simulink model "lab01_1"  (R2025a)
settings: Solver=VariableStepAuto  StartTime=0.0  StopTime=10  RelTol=1e-3
settings Model: Creator=grigorijtomczuk  LastModifiedBy=grigorijtomczuk

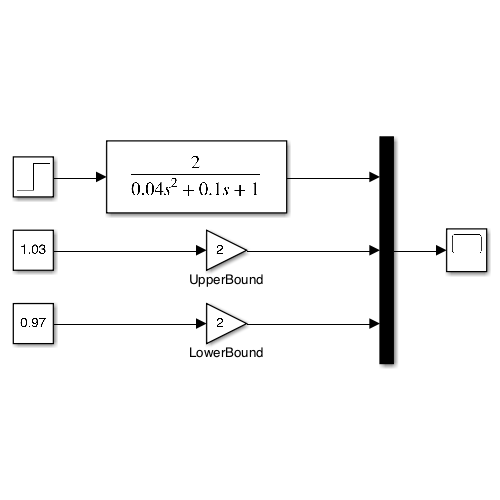
[thumbnail: Simulink's stored preview of the top-level diagram]
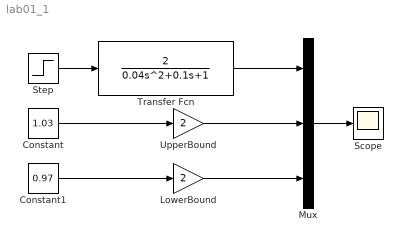
== system lab01_1 ==
  Constant : Constant  Value=1.03
  Constant1 : Constant  Value=0.97
  LowerBound : Gain  Gain=2
  Mux : Mux  Inputs=3
  Scope : Scope
      settings: ActiveDisplayYMinimum=-0.35929013888602573  ActiveDisplayYMaximum=3.2336112499742322
  Step : Step  SampleTime=0
  Transfer Fcn : TransferFcn  Numerator=[2]  Denominator=[0.04 0.1 1]
  UpperBound : Gain  Gain=2
  wires:
  Constant/1 -> UpperBound/1
  Constant1/1 -> LowerBound/1
  Step/1 -> Transfer Fcn/1
  Transfer Fcn/1 -> Mux/1
  UpperBound/1 -> Mux/2
  LowerBound/1 -> Mux/3
  Mux/1 -> Scope/1
